simulink model "controlGPI_pos_6dof_conMI"  (R2023b)
settings: Solver=ode45  StartTime=0.0  StopTime=tsim  FixedStep=1e-4  MaxStep=tstep
undefined symbols (not defined in the file): contr_robot_params, ddq, dq, MI_Contr1, MI_Contr2, MI_Contr3, MI_Contr4, MI_Contr5, MI_Contr6, MI_motor1, MI_motor2, MI_motor3, MI_motor4, MI_motor5, MI_motor6, ndof, NN_Bspline_params, NN_RBF_params, nn_select, ns, Pc, q0, q_cero, q_eq, robot_params, sigbuilder_block, t_qeq_init, t_tr_init, t_trtr, tau_L, tau_L_mags, tr_muestra, tr_ref, Wc, Zc
libraries: mcbcontrolslib x12, spsRMSLib x12, simulink x2
(part 4 of 4)

== system controlGPI_pos_6dof_conMI/Actuadores (Motores de inducción)/MI3 + PBC Torque Controller/Controlador PBC/Ley de control ==
  i_Sref : Inport
  d_iSref : Inport  Port=2
  psi_Rref : Inport  Port=3
  w_R : Inport  Port=4
  e_iS : Inport  Port=5
  Bus Selector : BusSelector  OutputSignals=epsilon_KiS
  K_iS : MATLAB Function  TreatAsAtomicUnit=on
  Ley de control : MATLAB Function  TreatAsAtomicUnit=on
  Scope17 : Scope
  U_S : Outport
  wires:
  [K_iS] -> Ley de control/7(Ki_s)
  d_iSref/1 -> Ley de control/3(d_iSref)
  psi_Rref/1 -> Ley de control/4(psi_Rref)
  i_Sref/1 -> Ley de control/2(i_Sref)
  Ley de control/1(u_S) -> U_S/1
  w_R/1 -> [w_R], Ley de control/5(w_R)
  e_iS/1 -> Ley de control/6(e_is)
  Bus Selector/1 -> K_iS/3(epsilon)  "<epsilon_KiS>"
  K_iS/1(K_iS) -> Scope17/1, [K_iS]
  [w_R] -> K_iS/2(w_R)
  [MI_motor_params] -> Ley de control/1(MI_motor_params)
  [MI_motor_params] -> K_iS/1(MI_motor_params)
  [PBC_params] -> Bus Selector/1

== system controlGPI_pos_6dof_conMI/Actuadores (Motores de inducción)/MI3 + PBC Torque Controller/Controlador PBC/Rampa+Ret ==
  Demux : Demux  Tag=STV Demux  Outputs=1
      settings: DisplayOption=none
  FromWs : FromWorkspace  Tag=STV FromWs  VariableName=tuvar
      SigBuilderData=|
      | common.afterFinalStr = 'Extrapolate'
      | common.sampleTime = 0
      | dataSet.timeRange = [0 20]
      | dataSet.name = 'Group 1'
      | sbobj.Groups.Name = 'Group 1'
      | sbobj.Groups.Signals.Name = 'Signal 1'
      | sbobj.Groups.Signals.XData = [0 0.5 1 20]
      | sbobj.Groups.Signals.YData = [0 0 0.64 0.64]
      | sbobj.Groups.TimeRange = [0 20]
  Signal 1 : Outport  Tag=STV Outport
  wires:
  Demux/1 -> Signal 1/1
  FromWs/1 -> Demux/1

== system controlGPI_pos_6dof_conMI/Actuadores (Motores de inducción)/MI3 + PBC Torque Controller/Controlador PBC/derivada Corrientes deseadas ==
  psi_Rref : Inport
  dpsi_Rref : Inport  Port=2
  psi_Rmagref : Inport  Port=3
  dpsi_Rmagref : Inport  Port=4
  ddpsi_Rmagref : Inport  Port=5
  tau_Rref : Inport  Port=6
  dtau_Rref : Inport  Port=7
  Scope10 : Scope
  derivada Corrientes deseadas : MATLAB Function  TreatAsAtomicUnit=on
  d_iSref : Outport
  wires:
  dpsi_Rref/1 -> derivada Corrientes deseadas/3(dpsi_Rref)
  tau_Rref/1 -> derivada Corrientes deseadas/7(tau_Rref)
  dtau_Rref/1 -> derivada Corrientes deseadas/8(dtau_Rref)
  dpsi_Rmagref/1 -> derivada Corrientes deseadas/5(dpsi_Rmagref)
  derivada Corrientes deseadas/1(d_iSref) -> Scope10/1, d_iSref/1
  psi_Rmagref/1 -> derivada Corrientes deseadas/4(psi_Rmagref)
  psi_Rref/1 -> derivada Corrientes deseadas/2(psi_Rref)
  ddpsi_Rmagref/1 -> derivada Corrientes deseadas/6(ddpsi_Rmagref)
  [MI_motor_params] -> derivada Corrientes deseadas/1(MI_motor_params)

== system controlGPI_pos_6dof_conMI/Actuadores (Motores de inducción)/MI4 + PBC Torque Controller/Controlador PBC/2 a 2(1) ==
  In1 : Inport
  In2 : Inport  Port=2
  Demux1 : Demux  Outputs=2
  Demux2 : Demux  Outputs=2
  Mux : Mux  Inputs=2
  Mux1 : Mux  Inputs=2
  Out1 : Outport
  Out2 : Outport  Port=2
  wires:
  Demux2/1 -> Mux/2
  Mux/1 -> Out1/1
  In2/1 -> Demux2/1
  In1/1 -> Demux1/1
  Demux1/1 -> Mux/1
  Demux1/2 -> Mux1/1
  Mux1/1 -> Out2/1
  Demux2/2 -> Mux1/2

== system controlGPI_pos_6dof_conMI/Actuadores (Motores de inducción)/MI4 + PBC Torque Controller/Controlador PBC/Corrientes y Flujos deseados ==
  w_R : Inport
  psi_Rref : Inport  Port=2
  tau_Rref : Inport  Port=3
  psi_Rmagref : Inport  Port=4
  dpsi_Rmagref1 : Inport  Port=5
  Corrientes/Flujos deseados : MATLAB Function  TreatAsAtomicUnit=on
  i_Sref : Outport
  dpsi_Rref : Outport  Port=2
  wires:
  tau_Rref/1 -> Corrientes/Flujos deseados/4(tau_Rref)
  Corrientes/Flujos deseados/1(i_Sref) -> i_Sref/1
  psi_Rref/1 -> Corrientes/Flujos deseados/3(psi_Rref)
  w_R/1 -> Corrientes/Flujos deseados/2(w_R)
  Corrientes/Flujos deseados/2(dpsi_Rref) -> dpsi_Rref/1
  psi_Rmagref/1 -> Corrientes/Flujos deseados/5(psi_Rmagref)
  dpsi_Rmagref1/1 -> Corrientes/Flujos deseados/6(dpsi_Rmagref)
  [MI_motor_params] -> Corrientes/Flujos deseados/1(MI_motor_params)

== system controlGPI_pos_6dof_conMI/Actuadores (Motores de inducción)/MI4 + PBC Torque Controller/Controlador PBC/Ley de control ==
  i_Sref : Inport
  d_iSref : Inport  Port=2
  psi_Rref : Inport  Port=3
  w_R : Inport  Port=4
  e_iS : Inport  Port=5
  Bus Selector : BusSelector  OutputSignals=epsilon_KiS
  K_iS : MATLAB Function  TreatAsAtomicUnit=on
  Ley de control : MATLAB Function  TreatAsAtomicUnit=on
  Scope17 : Scope
  U_S : Outport
  wires:
  [K_iS] -> Ley de control/7(Ki_s)
  d_iSref/1 -> Ley de control/3(d_iSref)
  psi_Rref/1 -> Ley de control/4(psi_Rref)
  i_Sref/1 -> Ley de control/2(i_Sref)
  Ley de control/1(u_S) -> U_S/1
  w_R/1 -> [w_R], Ley de control/5(w_R)
  e_iS/1 -> Ley de control/6(e_is)
  Bus Selector/1 -> K_iS/3(epsilon)  "<epsilon_KiS>"
  K_iS/1(K_iS) -> Scope17/1, [K_iS]
  [w_R] -> K_iS/2(w_R)
  [MI_motor_params] -> Ley de control/1(MI_motor_params)
  [MI_motor_params] -> K_iS/1(MI_motor_params)
  [PBC_params] -> Bus Selector/1

== system controlGPI_pos_6dof_conMI/Actuadores (Motores de inducción)/MI4 + PBC Torque Controller/Controlador PBC/Rampa+Ret ==
  Demux : Demux  Tag=STV Demux  Outputs=1
      settings: DisplayOption=none
  FromWs : FromWorkspace  Tag=STV FromWs  VariableName=tuvar
      SigBuilderData=|
      | common.afterFinalStr = 'Extrapolate'
      | common.sampleTime = 0
      | dataSet.timeRange = [0 20]
      | dataSet.name = 'Group 1'
      | sbobj.Groups.Name = 'Group 1'
      | sbobj.Groups.Signals.Name = 'Signal 1'
      | sbobj.Groups.Signals.XData = [0 0.5 1 20]
      | sbobj.Groups.Signals.YData = [0 0 0.64 0.64]
      | sbobj.Groups.TimeRange = [0 20]
  Signal 1 : Outport  Tag=STV Outport
  wires:
  Demux/1 -> Signal 1/1
  FromWs/1 -> Demux/1

== system controlGPI_pos_6dof_conMI/Actuadores (Motores de inducción)/MI4 + PBC Torque Controller/Controlador PBC/derivada Corrientes deseadas ==
  psi_Rref : Inport
  dpsi_Rref : Inport  Port=2
  psi_Rmagref : Inport  Port=3
  dpsi_Rmagref : Inport  Port=4
  ddpsi_Rmagref : Inport  Port=5
  tau_Rref : Inport  Port=6
  dtau_Rref : Inport  Port=7
  Scope10 : Scope
  derivada Corrientes deseadas : MATLAB Function  TreatAsAtomicUnit=on
  d_iSref : Outport
  wires:
  dpsi_Rref/1 -> derivada Corrientes deseadas/3(dpsi_Rref)
  tau_Rref/1 -> derivada Corrientes deseadas/7(tau_Rref)
  dtau_Rref/1 -> derivada Corrientes deseadas/8(dtau_Rref)
  dpsi_Rmagref/1 -> derivada Corrientes deseadas/5(dpsi_Rmagref)
  derivada Corrientes deseadas/1(d_iSref) -> Scope10/1, d_iSref/1
  psi_Rmagref/1 -> derivada Corrientes deseadas/4(psi_Rmagref)
  psi_Rref/1 -> derivada Corrientes deseadas/2(psi_Rref)
  ddpsi_Rmagref/1 -> derivada Corrientes deseadas/6(ddpsi_Rmagref)
  [MI_motor_params] -> derivada Corrientes deseadas/1(MI_motor_params)

== system controlGPI_pos_6dof_conMI/Actuadores (Motores de inducción)/MI5 + PBC Torque Controller/Controlador PBC/2 a 2(1) ==
  In1 : Inport
  In2 : Inport  Port=2
  Demux1 : Demux  Outputs=2
  Demux2 : Demux  Outputs=2
  Mux : Mux  Inputs=2
  Mux1 : Mux  Inputs=2
  Out1 : Outport
  Out2 : Outport  Port=2
  wires:
  Demux2/1 -> Mux/2
  Mux/1 -> Out1/1
  In2/1 -> Demux2/1
  In1/1 -> Demux1/1
  Demux1/1 -> Mux/1
  Demux1/2 -> Mux1/1
  Mux1/1 -> Out2/1
  Demux2/2 -> Mux1/2

== system controlGPI_pos_6dof_conMI/Actuadores (Motores de inducción)/MI5 + PBC Torque Controller/Controlador PBC/Corrientes y Flujos deseados ==
  w_R : Inport
  psi_Rref : Inport  Port=2
  tau_Rref : Inport  Port=3
  psi_Rmagref : Inport  Port=4
  dpsi_Rmagref1 : Inport  Port=5
  Corrientes/Flujos deseados : MATLAB Function  TreatAsAtomicUnit=on
  i_Sref : Outport
  dpsi_Rref : Outport  Port=2
  wires:
  tau_Rref/1 -> Corrientes/Flujos deseados/4(tau_Rref)
  Corrientes/Flujos deseados/1(i_Sref) -> i_Sref/1
  psi_Rref/1 -> Corrientes/Flujos deseados/3(psi_Rref)
  w_R/1 -> Corrientes/Flujos deseados/2(w_R)
  Corrientes/Flujos deseados/2(dpsi_Rref) -> dpsi_Rref/1
  psi_Rmagref/1 -> Corrientes/Flujos deseados/5(psi_Rmagref)
  dpsi_Rmagref1/1 -> Corrientes/Flujos deseados/6(dpsi_Rmagref)
  [MI_motor_params] -> Corrientes/Flujos deseados/1(MI_motor_params)

== system controlGPI_pos_6dof_conMI/Actuadores (Motores de inducción)/MI5 + PBC Torque Controller/Controlador PBC/Ley de control ==
  i_Sref : Inport
  d_iSref : Inport  Port=2
  psi_Rref : Inport  Port=3
  w_R : Inport  Port=4
  e_iS : Inport  Port=5
  Bus Selector : BusSelector  OutputSignals=epsilon_KiS
  K_iS : MATLAB Function  TreatAsAtomicUnit=on
  Ley de control : MATLAB Function  TreatAsAtomicUnit=on
  Scope17 : Scope
  U_S : Outport
  wires:
  [K_iS] -> Ley de control/7(Ki_s)
  d_iSref/1 -> Ley de control/3(d_iSref)
  psi_Rref/1 -> Ley de control/4(psi_Rref)
  i_Sref/1 -> Ley de control/2(i_Sref)
  Ley de control/1(u_S) -> U_S/1
  w_R/1 -> [w_R], Ley de control/5(w_R)
  e_iS/1 -> Ley de control/6(e_is)
  Bus Selector/1 -> K_iS/3(epsilon)  "<epsilon_KiS>"
  K_iS/1(K_iS) -> Scope17/1, [K_iS]
  [w_R] -> K_iS/2(w_R)
  [MI_motor_params] -> Ley de control/1(MI_motor_params)
  [MI_motor_params] -> K_iS/1(MI_motor_params)
  [PBC_params] -> Bus Selector/1

== system controlGPI_pos_6dof_conMI/Actuadores (Motores de inducción)/MI5 + PBC Torque Controller/Controlador PBC/Rampa+Ret ==
  Demux : Demux  Tag=STV Demux  Outputs=1
      settings: DisplayOption=none
  FromWs : FromWorkspace  Tag=STV FromWs  VariableName=tuvar
      SigBuilderData=|
      | common.afterFinalStr = 'Extrapolate'
      | common.sampleTime = 0
      | dataSet.timeRange = [0 20]
      | dataSet.name = 'Group 1'
      | sbobj.Groups.Name = 'Group 1'
      | sbobj.Groups.Signals.Name = 'Signal 1'
      | sbobj.Groups.Signals.XData = [0 0.5 1 20]
      | sbobj.Groups.Signals.YData = [0 0 0.64 0.64]
      | sbobj.Groups.TimeRange = [0 20]
  Signal 1 : Outport  Tag=STV Outport
  wires:
  Demux/1 -> Signal 1/1
  FromWs/1 -> Demux/1

== system controlGPI_pos_6dof_conMI/Actuadores (Motores de inducción)/MI5 + PBC Torque Controller/Controlador PBC/derivada Corrientes deseadas ==
  psi_Rref : Inport
  dpsi_Rref : Inport  Port=2
  psi_Rmagref : Inport  Port=3
  dpsi_Rmagref : Inport  Port=4
  ddpsi_Rmagref : Inport  Port=5
  tau_Rref : Inport  Port=6
  dtau_Rref : Inport  Port=7
  Scope10 : Scope
  derivada Corrientes deseadas : MATLAB Function  TreatAsAtomicUnit=on
  d_iSref : Outport
  wires:
  dpsi_Rref/1 -> derivada Corrientes deseadas/3(dpsi_Rref)
  tau_Rref/1 -> derivada Corrientes deseadas/7(tau_Rref)
  dtau_Rref/1 -> derivada Corrientes deseadas/8(dtau_Rref)
  dpsi_Rmagref/1 -> derivada Corrientes deseadas/5(dpsi_Rmagref)
  derivada Corrientes deseadas/1(d_iSref) -> Scope10/1, d_iSref/1
  psi_Rmagref/1 -> derivada Corrientes deseadas/4(psi_Rmagref)
  psi_Rref/1 -> derivada Corrientes deseadas/2(psi_Rref)
  ddpsi_Rmagref/1 -> derivada Corrientes deseadas/6(ddpsi_Rmagref)
  [MI_motor_params] -> derivada Corrientes deseadas/1(MI_motor_params)

== system controlGPI_pos_6dof_conMI/Actuadores (Motores de inducción)/MI6 + PBC Torque Controller/Controlador PBC/2 a 2(1) ==
  In1 : Inport
  In2 : Inport  Port=2
  Demux1 : Demux  Outputs=2
  Demux2 : Demux  Outputs=2
  Mux : Mux  Inputs=2
  Mux1 : Mux  Inputs=2
  Out1 : Outport
  Out2 : Outport  Port=2
  wires:
  Demux2/1 -> Mux/2
  Mux/1 -> Out1/1
  In2/1 -> Demux2/1
  In1/1 -> Demux1/1
  Demux1/1 -> Mux/1
  Demux1/2 -> Mux1/1
  Mux1/1 -> Out2/1
  Demux2/2 -> Mux1/2

== system controlGPI_pos_6dof_conMI/Actuadores (Motores de inducción)/MI6 + PBC Torque Controller/Controlador PBC/Corrientes y Flujos deseados ==
  w_R : Inport
  psi_Rref : Inport  Port=2
  tau_Rref : Inport  Port=3
  psi_Rmagref : Inport  Port=4
  dpsi_Rmagref1 : Inport  Port=5
  Corrientes/Flujos deseados : MATLAB Function  TreatAsAtomicUnit=on
  i_Sref : Outport
  dpsi_Rref : Outport  Port=2
  wires:
  tau_Rref/1 -> Corrientes/Flujos deseados/4(tau_Rref)
  Corrientes/Flujos deseados/1(i_Sref) -> i_Sref/1
  psi_Rref/1 -> Corrientes/Flujos deseados/3(psi_Rref)
  w_R/1 -> Corrientes/Flujos deseados/2(w_R)
  Corrientes/Flujos deseados/2(dpsi_Rref) -> dpsi_Rref/1
  psi_Rmagref/1 -> Corrientes/Flujos deseados/5(psi_Rmagref)
  dpsi_Rmagref1/1 -> Corrientes/Flujos deseados/6(dpsi_Rmagref)
  [MI_motor_params] -> Corrientes/Flujos deseados/1(MI_motor_params)

== system controlGPI_pos_6dof_conMI/Actuadores (Motores de inducción)/MI6 + PBC Torque Controller/Controlador PBC/Ley de control ==
  i_Sref : Inport
  d_iSref : Inport  Port=2
  psi_Rref : Inport  Port=3
  w_R : Inport  Port=4
  e_iS : Inport  Port=5
  Bus Selector : BusSelector  OutputSignals=epsilon_KiS
  K_iS : MATLAB Function  TreatAsAtomicUnit=on
  Ley de control : MATLAB Function  TreatAsAtomicUnit=on
  Scope17 : Scope
  U_S : Outport
  wires:
  [K_iS] -> Ley de control/7(Ki_s)
  d_iSref/1 -> Ley de control/3(d_iSref)
  psi_Rref/1 -> Ley de control/4(psi_Rref)
  i_Sref/1 -> Ley de control/2(i_Sref)
  Ley de control/1(u_S) -> U_S/1
  w_R/1 -> [w_R], Ley de control/5(w_R)
  e_iS/1 -> Ley de control/6(e_is)
  Bus Selector/1 -> K_iS/3(epsilon)  "<epsilon_KiS>"
  K_iS/1(K_iS) -> Scope17/1, [K_iS]
  [w_R] -> K_iS/2(w_R)
  [MI_motor_params] -> Ley de control/1(MI_motor_params)
  [MI_motor_params] -> K_iS/1(MI_motor_params)
  [PBC_params] -> Bus Selector/1

== system controlGPI_pos_6dof_conMI/Actuadores (Motores de inducción)/MI6 + PBC Torque Controller/Controlador PBC/Rampa+Ret ==
  Demux : Demux  Tag=STV Demux  Outputs=1
      settings: DisplayOption=none
  FromWs : FromWorkspace  Tag=STV FromWs  VariableName=tuvar
      SigBuilderData=|
      | common.afterFinalStr = 'Extrapolate'
      | common.sampleTime = 0
      | dataSet.timeRange = [0 20]
      | dataSet.name = 'Group 1'
      | sbobj.Groups.Name = 'Group 1'
      | sbobj.Groups.Signals.Name = 'Signal 1'
      | sbobj.Groups.Signals.XData = [0 0.5 1 20]
      | sbobj.Groups.Signals.YData = [0 0 0.64 0.64]
      | sbobj.Groups.TimeRange = [0 20]
  Signal 1 : Outport  Tag=STV Outport
  wires:
  Demux/1 -> Signal 1/1
  FromWs/1 -> Demux/1

== system controlGPI_pos_6dof_conMI/Actuadores (Motores de inducción)/MI6 + PBC Torque Controller/Controlador PBC/derivada Corrientes deseadas ==
  psi_Rref : Inport
  dpsi_Rref : Inport  Port=2
  psi_Rmagref : Inport  Port=3
  dpsi_Rmagref : Inport  Port=4
  ddpsi_Rmagref : Inport  Port=5
  tau_Rref : Inport  Port=6
  dtau_Rref : Inport  Port=7
  Scope10 : Scope
  derivada Corrientes deseadas : MATLAB Function  TreatAsAtomicUnit=on
  d_iSref : Outport
  wires:
  dpsi_Rref/1 -> derivada Corrientes deseadas/3(dpsi_Rref)
  tau_Rref/1 -> derivada Corrientes deseadas/7(tau_Rref)
  dtau_Rref/1 -> derivada Corrientes deseadas/8(dtau_Rref)
  dpsi_Rmagref/1 -> derivada Corrientes deseadas/5(dpsi_Rmagref)
  derivada Corrientes deseadas/1(d_iSref) -> Scope10/1, d_iSref/1
  psi_Rmagref/1 -> derivada Corrientes deseadas/4(psi_Rmagref)
  psi_Rref/1 -> derivada Corrientes deseadas/2(psi_Rref)
  ddpsi_Rmagref/1 -> derivada Corrientes deseadas/6(ddpsi_Rmagref)
  [MI_motor_params] -> derivada Corrientes deseadas/1(MI_motor_params)

== matlab function controlGPI_pos_6dof_conMI/ControladorGPI + NN/Ley de control ==
  data: robot_din input; v output size=[6,1]; eqB5 input size=[6,1]; eqB4 input size=[6,1]; eqB3 input size=[6,1]; eqB2 input size=[6,1]; eqB1 input size=[6,1]; tau_R output size=[6,1]
function [v,tau_R] = fcn(robot_din,eqB5,eqB4,eqB3,eqB2,eqB1)

D = robot_din.D;

v = - eqB5 - eqB4 - eqB3 - eqB2 - eqB1;

tau_R = D*v;

== matlab function controlGPI_pos_6dof_conMI/ControladorGPI + NN/Matriz de parámetros B ==
  data: B5 output size=[6,1]; B4 output size=[6,1]; B3 output size=[6,1]; B2 output size=[6,1]; Zc input size=[6,1]; B1 output size=[6,1]; Wc input size=[6,1]; Pc input size=[6,1]
function [B5,B4,B3,B2,B1] = fcn(Zc,Wc,Pc)

B = zeros(6,6);

B(:,1) = Wc.^4.*Pc;
B(:,2) = 4*Wc.^3.*Zc.*Pc + Wc.^4;
B(:,3) = 4*Wc.^3.*Zc + 4*Wc.^2.*Zc.^2.*Pc + 2.*Wc.^2.*Pc;
B(:,4) = 2*Wc.^2 + 4*Wc.^2.*Zc.^2 + 4*Wc.*Zc.*Pc;
B(:,5) = 4*Wc.*Zc + Pc;
% B(:,6) = ones(3,6);

B1 = B(:,1);
B2 = B(:,2);
B3 = B(:,3);
B4 = B(:,4);
B5 = B(:,5);
% B6 = B(:,6);

== matlab function controlGPI_pos_6dof_conMI/ControladorGPI + NN/Red neuronal/B-Spline NNs/Red Neuronal B-spline ==
  data: NN_Bspline_params input; e_q input size=[6,1]; Wc output size=[6,1]; Zc output size=[6,1]; Pc output size=[6,1]; e_px input size=[6,1]; e_py input size=[6,1]; e_pz input size=[6,1]; newweightsWc output; newweightsZc output; newweightsPc output; weightsWc input; weightsZc input; weightsPc input
function [Wc, Zc, Pc, newweightsWc, newweightsZc, newweightsPc]   = BSpline_NN(NN_Bspline_params,e_q,e_px,e_py,e_pz,weightsWc,weightsZc,weightsPc)

deltaWc = NN_Bspline_params.delta.deltaWc;
deltaZc = NN_Bspline_params.delta.deltaZc;
deltaPc = NN_Bspline_params.delta.deltaPc;

lambdaWc = NN_Bspline_params.lambda.lambdaWc;
lambdaZc = NN_Bspline_params.lambda.lambdaZc;
lambdaPc = NN_Bspline_params.lambda.lambdaPc;

if NN_Bspline_params.num_inputs == 1
    nn_inputs = e_q;
elseif NN_Bspline_params.num_inputs == 4
    nn_inputs = [e_q,e_px,e_py,e_pz];
else
    nn_inputs = e_q;
end

delta = [deltaWc;
         deltaZc;
         deltaPc];

lambda = cat(1,lambdaWc,lambdaZc,lambdaPc);
weights = cat(1,weightsWc,weightsZc,weightsPc);

[newparams,newweights] = NN_Bspline.Gradient_Descent(delta,weights,lambda,nn_inputs);

Wc = newparams(1,:)';
Zc = newparams(2,:)';
Pc = newparams(3,:)';

newweightsWc = newweights(1,:,:);
newweightsZc = newweights(2,:,:);
newweightsPc = newweights(3,:,:);

end

== matlab function controlGPI_pos_6dof_conMI/ControladorGPI + NN/Red neuronal/RBF NNs/Red Neuronal RBF ==
  data: NN_RBF_params input; e_q input size=[6,1]; Wc output size=[6,1]; Zc output size=[6,1]; Pc output size=[6,1]; e_px input size=[6,1]; e_py input size=[6,1]; e_pz input size=[6,1]; weightsWc output; weightsZc output; weightsPc output; weightsWc input; weightsZc input; weightsPc input
function [Wc, Zc, Pc, weightsWc, weightsZc, weightsPc] = RBF_NN(NN_RBF_params,e_q,e_px,e_py,e_pz, weightsWc, weightsZc, weightsPc)

%k = NN_RBF_params.rbf_params.k;
centers = NN_RBF_params.rbf_params.C';
radius = NN_RBF_params.rbf_params.sigma;

deltaWc = NN_RBF_params.delta.deltaWc;
deltaZc = NN_RBF_params.delta.deltaZc;
deltaPc = NN_RBF_params.delta.deltaPc;

if NN_RBF_params.num_inputs == 1
    NNRBF_inputs = e_q;
elseif NN_RBF_params.num_inputs == 4
    NNRBF_inputs = [e_q,e_px,e_py,e_pz];
else
    NNRBF_inputs = e_q;
end

delta = [deltaWc;
         deltaZc;
         deltaPc];

weights = cat(1,weightsWc,weightsZc,weightsPc);

[newparams,newweights] = NN_RBF.Gradient_Descent(delta,weights,centers,radius,NNRBF_inputs);

Wc = newparams(1,:)';
Zc = newparams(2,:)';
Pc = newparams(3,:)';

weightsWc = newweights(1,:,:);
weightsZc = newweights(2,:,:);
weightsPc = newweights(3,:,:);

end

== matlab function controlGPI_pos_6dof_conMI/Perfil torque de carga tau_L/If Action Subsystem/Polinomio 7mo orden sen ==
  data: t input; perfil_params input; qpol output; vpol output; apol output; jpol output
function [qpol,vpol,apol,jpol] = fcn(t,perfil_params)

%Trayectoria de referencia

q0 = 0;
q1 = perfil_params.senoidal.amplitud;

% v0 = perfil_params.polinomio7.vel.inicial;
% v1 = perfil_params.polinomio7.vel.final;
% 
% ac0 = perfil_params.polinomio7.acel.inicial;
% ac1 = perfil_params.polinomio7.acel.final;
% 
% j0 = perfil_params.polinomio7.jerk.inicial;
% j1 = perfil_params.polinomio7.jerk.inicial;

if perfil_params.senoidal.tiempo_inicio-1>0
    t0 = perfil_params.senoidal.tiempo_inicio-1;
else
    t0 = 0;
end
t1 = perfil_params.senoidal.tiempo_inicio;

% Coeficientes de un polinomio de 7mo grado
[qpol,vpol,apol,jpol] = pol7(t,q1,q0,t0,t1);

== matlab function controlGPI_pos_6dof_conMI/Perfil torque de carga tau_L/If Action Subsystem4/Polinomio 7mo orden tau_L ==
  data: t input; perfil_params input; qpol output; vpol output; apol output; jpol output
function [qpol,vpol,apol,jpol] = fcn(t,perfil_params)

%Trayectoria de referencia

q0 = perfil_params.polinomio7.pos.inicial;
q1 = perfil_params.polinomio7.pos.final;

% v0 = perfil_params.polinomio7.vel.inicial;
% v1 = perfil_params.polinomio7.vel.final;
% 
% ac0 = perfil_params.polinomio7.acel.inicial;
% ac1 = perfil_params.polinomio7.acel.final;
% 
% j0 = perfil_params.polinomio7.jerk.inicial;
% j1 = perfil_params.polinomio7.jerk.inicial;

t0 = perfil_params.polinomio7.tiempo.inicial;
t1 = perfil_params.polinomio7.tiempo.final;

% Coeficientes de un polinomio de 7mo grado
[qpol,vpol,apol,jpol] = pol7(t,q0,q1,t0,t1);

== matlab function controlGPI_pos_6dof_conMI/Perfil torque de carga tau_L/If Action Subsystem7/Trayectoria 15 segmentos ==
  data: t input size=1; q output size=1; perfil_params input
function q = fcn(t,perfil_params)

q0 = perfil_params.tr15segs.pos.inicial;
q1 = perfil_params.tr15segs.pos.final;

t0 = perfil_params.tr15segs.tiempo.inicial;

vel_path = perfil_params.tr15segs.vel_path;
acel_path = perfil_params.tr15segs.acel_path;
snap_path = perfil_params.tr15segs.snap_path;

dist = norm(q1-q0);
num_steps = 1000;




[interq,T] = pol15segs.bounded_tr(dist,num_steps,vel_path,acel_path,snap_path,0);

tstep = T/num_steps;
t1 = t0 + T;
t_tr = (t0:tstep:t1)';


[~,idt] = min(t_tr-t);
dire = (q1 - q0)/dist;
q = q0 + dire*interq(idt);

== matlab function controlGPI_pos_6dof_conMI/ISCI ==
  data: tau input; ISCI output
function ISCI = fcn(tau)

ISCI = tau.^2;

== matlab function controlGPI_pos_6dof_conMI/Perfil torque de carga tau_L/If Action Subsystem6/Polinomio 7mo orden timeseries ==
  data: t input; qpol output; vpol output; apol output; jpol output
function [qpol,vpol,apol,jpol] = fcn(t)

q0 = 0;
q1 = 1;

t0 = 0.5;
t1 = 1;

%Trayectoria de referencia

% Coeficientes de un polinomio de 7mo grado
[qpol,vpol,apol,jpol] = pol7(t,q0,q1,t0,t1);

== matlab function controlGPI_pos_6dof_conMI/Actuadores (Motores de inducción)/MI3 + PBC Torque Controller/Calculo de Potencia eléctrica/ab0 - ABC1 ==
  data: BPu input size=[2,1]; u output size=[3,1]
function u = fcn(BPu)

BPu = vertcat(BPu,0);

% Power invariant
BP = transforms.Clarke_transform(1);

u = BP^-1*BPu;

== matlab function controlGPI_pos_6dof_conMI/Perfil torque de carga tau_L/If Action Subsystem5/Tren de esca ==
  data: t input; q output; perfil_params input
function q = fcn(t,perfil_params)

q = Perfil_trayectoria.trEsca(t,perfil_params);

== matlab function controlGPI_pos_6dof_conMI/ITAE ==
  data: t input; ITAE output; eq input
function ITAE = fcn(t,eq)

ITAE = t.*abs(eq);

== matlab function controlGPI_pos_6dof_conMI/Actuadores (Motores de inducción)/MI2 + PBC Torque Controller/Calculo de Potencia eléctrica/ab0 - ABC ==
  data: BPu input size=[2,1]; u output size=[3,1]
function u = fcn(BPu)

BPu = vertcat(BPu,0);

% Power invariant
BP = transforms.Clarke_transform(1);

u = BP^-1*BPu;

== matlab function controlGPI_pos_6dof_conMI/Actuadores (Motores de inducción)/MI2 + PBC Torque Controller/Calculo de Potencia eléctrica/ab0 - ABC1 ==
  data: BPu input size=[2,1]; u output size=[3,1]
function u = fcn(BPu)

BPu = vertcat(BPu,0);

% Power invariant
BP = transforms.Clarke_transform(1);

u = BP^-1*BPu;

== matlab function controlGPI_pos_6dof_conMI/Actuadores (Motores de inducción)/MI2 + PBC Torque Controller/Controlador PBC/Corrientes y Flujos deseados/Corrientes//Flujos deseados ==
  data: MI_motor_params input; w_R input; i_Sref output size=[2 1]; psi_Rref input size=[2,1]; tau_Rref input; psi_Rmagref input; dpsi_Rmagref input; dpsi_Rref output size=[2,1]
function [i_Sref,dpsi_Rref] = fcn(MI_motor_params,w_R,psi_Rref,tau_Rref,psi_Rmagref,dpsi_Rmagref)

i_Sref = PBC_Torque_Controller.i_Sref(MI_motor_params,psi_Rref,tau_Rref,psi_Rmagref,dpsi_Rmagref);
dpsi_Rref = PBC_Torque_Controller.dpsi_Ref(MI_motor_params,w_R,psi_Rref,tau_Rref,psi_Rmagref,dpsi_Rmagref);

== matlab function controlGPI_pos_6dof_conMI/Actuadores (Motores de inducción)/MI2 + PBC Torque Controller/Controlador PBC/Ley de control/K_iS ==
  data: MI_motor_params input; w_R input; epsilon input; K_iS output
function K_iS = fcn(MI_motor_params,w_R,epsilon)

K_iS = PBC_Torque_Controller.K_iS(MI_motor_params,w_R,epsilon);

== matlab function controlGPI_pos_6dof_conMI/Modelo robot manipulador (Dinámica directa)/Dinámica directa ==
  data: robot_params input; q input; ddq output size=[6,1]; dq input size=[6,1]; tau_R input size=[6,1]; tau_L input size=[6,1]
function ddq = fcn(robot_params,q,dq,tau_R,tau_L)

robot_din = robot_dinm.din_6dof(robot_params,q,dq);

D = robot_din.D;
C = robot_din.C;
G = robot_din.G;
g = robot_din.g;

ddq = D^-1*(-C*dq-G*g+(tau_R-tau_L));

== matlab function controlGPI_pos_6dof_conMI/Actuadores (Motores de inducción)/MI3 + PBC Torque Controller/Controlador PBC/Corrientes y Flujos deseados/Corrientes//Flujos deseados ==
  data: MI_motor_params input; w_R input; i_Sref output size=[2 1]; psi_Rref input size=[2,1]; tau_Rref input; psi_Rmagref input; dpsi_Rmagref input; dpsi_Rref output size=[2,1]
function [i_Sref,dpsi_Rref] = fcn(MI_motor_params,w_R,psi_Rref,tau_Rref,psi_Rmagref,dpsi_Rmagref)

i_Sref = PBC_Torque_Controller.i_Sref(MI_motor_params,psi_Rref,tau_Rref,psi_Rmagref,dpsi_Rmagref);
dpsi_Rref = PBC_Torque_Controller.dpsi_Ref(MI_motor_params,w_R,psi_Rref,tau_Rref,psi_Rmagref,dpsi_Rmagref);

== matlab function controlGPI_pos_6dof_conMI/Actuadores (Motores de inducción)/MI3 + PBC Torque Controller/Controlador PBC/Ley de control/K_iS ==
  data: MI_motor_params input; w_R input; epsilon input; K_iS output
function K_iS = fcn(MI_motor_params,w_R,epsilon)

K_iS = PBC_Torque_Controller.K_iS(MI_motor_params,w_R,epsilon);

== matlab function controlGPI_pos_6dof_conMI/Actuadores (Motores de inducción)/MI2 + PBC Torque Controller/Controlador PBC/Ley de control/Ley de control ==
  data: MI_motor_params input; i_Sref input size=[2,1]; d_iSref input size=[2,1]; u_S output size=[2 1]; psi_Rref input size=[2,1]; w_R input; e_is input; Ki_s input
function u_S = fcn(MI_motor_params,i_Sref,d_iSref,psi_Rref,w_R,e_is,Ki_s)

u_S = PBC_Torque_Controller.ley_control_uS(MI_motor_params,i_Sref,d_iSref,psi_Rref,w_R,e_is,Ki_s);

== matlab function controlGPI_pos_6dof_conMI/Actuadores (Motores de inducción)/MI1 + PBC Torque Controller/Controlador PBC/Corrientes y Flujos deseados/Corrientes//Flujos deseados ==
  data: MI_motor_params input; w_R input; i_Sref output size=[2 1]; psi_Rref input size=[2,1]; tau_Rref input; psi_Rmagref input; dpsi_Rmagref input; dpsi_Rref output size=[2,1]
function [i_Sref,dpsi_Rref] = fcn(MI_motor_params,w_R,psi_Rref,tau_Rref,psi_Rmagref,dpsi_Rmagref)

i_Sref = PBC_Torque_Controller.i_Sref(MI_motor_params,psi_Rref,tau_Rref,psi_Rmagref,dpsi_Rmagref);
dpsi_Rref = PBC_Torque_Controller.dpsi_Ref(MI_motor_params,w_R,psi_Rref,tau_Rref,psi_Rmagref,dpsi_Rmagref);

== matlab function controlGPI_pos_6dof_conMI/Actuadores (Motores de inducción)/MI1 + PBC Torque Controller/Controlador PBC/Ley de control/K_iS ==
  data: MI_motor_params input; w_R input; epsilon input; K_iS output
function K_iS = fcn(MI_motor_params,w_R,epsilon)

K_iS = PBC_Torque_Controller.K_iS(MI_motor_params,w_R,epsilon);

== matlab function controlGPI_pos_6dof_conMI/Trayectoria de referencia/Dinamica inversa (referencia) ==
  data: robot_params input; tau_s output size=[6,1]; q input size=[6,1]; dq input size=[6,1]; ddq input size=[6,1]
function tau_s = fcn(robot_params,q,dq,ddq)

robot_din = robot_dinm.din_6dof(robot_params,q,dq);

D = robot_din.D;
C = robot_din.C;
G = robot_din.G;
g = robot_din.g;

tau_s = D*ddq + C*dq + G*g;

== matlab function controlGPI_pos_6dof_conMI/Actuadores (Motores de inducción)/MI1 + PBC Torque Controller/Calculo de Potencia eléctrica/ab0 - ABC ==
  data: BPu input size=[2,1]; u output size=[3,1]
function u = fcn(BPu)

BPu = vertcat(BPu,0);

% Power invariant
BP = transforms.Clarke_transform(1);

u = BP^-1*BPu;

== matlab function controlGPI_pos_6dof_conMI/Actuadores (Motores de inducción)/MI1 + PBC Torque Controller/Controlador PBC/Ley de control/Ley de control ==
  data: MI_motor_params input; i_Sref input size=[2,1]; d_iSref input size=[2,1]; u_S output size=[2 1]; psi_Rref input size=[2,1]; w_R input; e_is input; Ki_s input
function u_S = fcn(MI_motor_params,i_Sref,d_iSref,psi_Rref,w_R,e_is,Ki_s)

u_S = PBC_Torque_Controller.ley_control_uS(MI_motor_params,i_Sref,d_iSref,psi_Rref,w_R,e_is,Ki_s);

== matlab function controlGPI_pos_6dof_conMI/Actuadores (Motores de inducción)/MI1 + PBC Torque Controller/Calculo de Potencia eléctrica/ab0 - ABC1 ==
  data: BPu input size=[2,1]; u output size=[3,1]
function u = fcn(BPu)

BPu = vertcat(BPu,0);

% Power invariant
BP = transforms.Clarke_transform(1);

u = BP^-1*BPu;

== matlab function controlGPI_pos_6dof_conMI/Actuadores (Motores de inducción)/MI3 + PBC Torque Controller/Controlador PBC/Ley de control/Ley de control ==
  data: MI_motor_params input; i_Sref input size=[2,1]; d_iSref input size=[2,1]; u_S output size=[2 1]; psi_Rref input size=[2,1]; w_R input; e_is input; Ki_s input
function u_S = fcn(MI_motor_params,i_Sref,d_iSref,psi_Rref,w_R,e_is,Ki_s)

u_S = PBC_Torque_Controller.ley_control_uS(MI_motor_params,i_Sref,d_iSref,psi_Rref,w_R,e_is,Ki_s);

== matlab function controlGPI_pos_6dof_conMI/Actuadores (Motores de inducción)/MI3 + PBC Torque Controller/Controlador PBC/derivada Corrientes deseadas/derivada Corrientes deseadas ==
  data: MI_motor_params input; d_iSref output size=[2 1]; psi_Rref input size=[2,1]; dpsi_Rref input size=[2,1]; psi_Rmagref input; dpsi_Rmagref input; ddpsi_Rmagref input; tau_Rref input; dtau_Rref input
function d_iSref = fcn(MI_motor_params,psi_Rref,dpsi_Rref,psi_Rmagref,dpsi_Rmagref,ddpsi_Rmagref,tau_Rref,dtau_Rref)

d_iSref = PBC_Torque_Controller.d_iSref(MI_motor_params,psi_Rref,dpsi_Rref,psi_Rmagref,dpsi_Rmagref,ddpsi_Rmagref,tau_Rref,dtau_Rref);

== matlab function controlGPI_pos_6dof_conMI/Actuadores (Motores de inducción)/MI3 + PBC Torque Controller/Modelo MI (Subsistema eléctrico)/Modelo Motor de inducción (Subsistema eléctrico) ==
  data: MI_motor_params input; di_Sab output double size=[2 1]; dpsi_Rab output double size=[2 1]; u_Sab input double size=[2 1]; i_Sab input double size=[2 1]; psi_Rab input double size=[2 1]; w_R input double size=1; tau_R output size=1; tau_L input
function [di_Sab,dpsi_Rab,tau_R] = fcn(MI_motor_params,u_Sab,i_Sab,psi_Rab,w_R,tau_L)

[di_Sab,dpsi_Rab,dw_R,tau_R] = MI_model.MI_space_state(MI_motor_params,u_Sab,i_Sab,psi_Rab,w_R,tau_L);

== matlab function controlGPI_pos_6dof_conMI/Actuadores (Motores de inducción)/MI1 + PBC Torque Controller/Controlador PBC/derivada Corrientes deseadas/derivada Corrientes deseadas ==
  data: MI_motor_params input; d_iSref output size=[2 1]; psi_Rref input size=[2,1]; dpsi_Rref input size=[2,1]; psi_Rmagref input; dpsi_Rmagref input; ddpsi_Rmagref input; tau_Rref input; dtau_Rref input
function d_iSref = fcn(MI_motor_params,psi_Rref,dpsi_Rref,psi_Rmagref,dpsi_Rmagref,ddpsi_Rmagref,tau_Rref,dtau_Rref)

d_iSref = PBC_Torque_Controller.d_iSref(MI_motor_params,psi_Rref,dpsi_Rref,psi_Rmagref,dpsi_Rmagref,ddpsi_Rmagref,tau_Rref,dtau_Rref);

== matlab function controlGPI_pos_6dof_conMI/Actuadores (Motores de inducción)/MI1 + PBC Torque Controller/Modelo MI (Subsistema eléctrico)/Modelo Motor de inducción (Subsistema eléctrico) ==
  data: MI_motor_params input; di_Sab output double size=[2 1]; dpsi_Rab output double size=[2 1]; u_Sab input double size=[2 1]; i_Sab input double size=[2 1]; psi_Rab input double size=[2 1]; w_R input double size=1; tau_R output size=1; tau_L input
function [di_Sab,dpsi_Rab,tau_R] = fcn(MI_motor_params,u_Sab,i_Sab,psi_Rab,w_R,tau_L)

[di_Sab,dpsi_Rab,dw_R,tau_R] = MI_model.MI_space_state(MI_motor_params,u_Sab,i_Sab,psi_Rab,w_R,tau_L);

== matlab function controlGPI_pos_6dof_conMI/Actuadores (Motores de inducción)/MI1 + PBC Torque Controller/Modelo MI (Subsistema eléctrico)/ab//dq ==
  data: psi_ra input; psi_Rmag output; psi_rb input; rho output
function [psi_Rmag,rho] = fcn(psi_ra,psi_rb)

psi_Rmag = sqrt(psi_ra^2+psi_rb^2);
rho = atan2(psi_rb,psi_ra);

== matlab function controlGPI_pos_6dof_conMI/Actuadores (Motores de inducción)/MI3 + PBC Torque Controller/Modelo MI (Subsistema eléctrico)/ab//dq ==
  data: psi_ra input; psi_Rmag output; psi_rb input; rho output
function [psi_Rmag,rho] = fcn(psi_ra,psi_rb)

psi_Rmag = sqrt(psi_ra^2+psi_rb^2);
rho = atan2(psi_rb,psi_ra);

== matlab function controlGPI_pos_6dof_conMI/Actuadores (Motores de inducción)/MI4 + PBC Torque Controller/Calculo de Potencia eléctrica/ab0 - ABC ==
  data: BPu input size=[2,1]; u output size=[3,1]
function u = fcn(BPu)

BPu = vertcat(BPu,0);

% Power invariant
BP = transforms.Clarke_transform(1);

u = BP^-1*BPu;

== matlab function controlGPI_pos_6dof_conMI/Actuadores (Motores de inducción)/MI4 + PBC Torque Controller/Calculo de Potencia eléctrica/ab0 - ABC1 ==
  data: BPu input size=[2,1]; u output size=[3,1]
function u = fcn(BPu)

BPu = vertcat(BPu,0);

% Power invariant
BP = transforms.Clarke_transform(1);

u = BP^-1*BPu;

== matlab function controlGPI_pos_6dof_conMI/Trayectoria de referencia/q to xyz (referencia) ==
  data: p output size=[3,6]; robot_params input; q input size=[6,1]
function p = fcn(robot_params,q)

p = robot_cin.cin_dirp_6dof(robot_params,q);

== matlab function controlGPI_pos_6dof_conMI/Trayectoria de referencia/xyz to q (referencia) ==
  data: robot_params input; q output size=[6,1]; r input size=[3,1]; dr input size=[3,1]; ddr input size=[3,1]; dq output size=[6,1]; ddq output size=[6,1]; R input size=[3,3]
function [q,dq,ddq] = fcn(robot_params,r,dr,ddr,R)

[q,dq,ddq] = robot_cin.cin_inv_6dof(robot_params,r,dr,ddr,R);

== matlab function controlGPI_pos_6dof_conMI/q to xyz (robot)/q to xyz (robot) ==
  data: p output size=[3,6]; robot_params input; q input size=[6,1]; dq input size=[6,1]; ddq input size=[6,1]; dp output size=[3,1]; ddp output size=[3,1]
function [p,dp,ddp] = fcn(robot_params,q,dq,ddq)

p = robot_cin.cin_dirp_6dof(robot_params,q);

JP = robot_cin.JP_6dof(robot_params,q);
dp = JP*dq;

dJP = robot_cin.dJP_6dof(robot_params,q,dq);
ddp = dJP*ddq;

== matlab function controlGPI_pos_6dof_conMI/Actuadores (Motores de inducción)/MI4 + PBC Torque Controller/Controlador PBC/Corrientes y Flujos deseados/Corrientes//Flujos deseados ==
  data: MI_motor_params input; w_R input; i_Sref output size=[2 1]; psi_Rref input size=[2,1]; tau_Rref input; psi_Rmagref input; dpsi_Rmagref input; dpsi_Rref output size=[2,1]
function [i_Sref,dpsi_Rref] = fcn(MI_motor_params,w_R,psi_Rref,tau_Rref,psi_Rmagref,dpsi_Rmagref)

i_Sref = PBC_Torque_Controller.i_Sref(MI_motor_params,psi_Rref,tau_Rref,psi_Rmagref,dpsi_Rmagref);
dpsi_Rref = PBC_Torque_Controller.dpsi_Ref(MI_motor_params,w_R,psi_Rref,tau_Rref,psi_Rmagref,dpsi_Rmagref);

== matlab function controlGPI_pos_6dof_conMI/Actuadores (Motores de inducción)/MI4 + PBC Torque Controller/Controlador PBC/Ley de control/K_iS ==
  data: MI_motor_params input; w_R input; epsilon input; K_iS output
function K_iS = fcn(MI_motor_params,w_R,epsilon)

K_iS = PBC_Torque_Controller.K_iS(MI_motor_params,w_R,epsilon);

== matlab function controlGPI_pos_6dof_conMI/Actuadores (Motores de inducción)/MI4 + PBC Torque Controller/Controlador PBC/Ley de control/Ley de control ==
  data: MI_motor_params input; i_Sref input size=[2,1]; d_iSref input size=[2,1]; u_S output size=[2 1]; psi_Rref input size=[2,1]; w_R input; e_is input; Ki_s input
function u_S = fcn(MI_motor_params,i_Sref,d_iSref,psi_Rref,w_R,e_is,Ki_s)

u_S = PBC_Torque_Controller.ley_control_uS(MI_motor_params,i_Sref,d_iSref,psi_Rref,w_R,e_is,Ki_s);

== matlab function controlGPI_pos_6dof_conMI/Actuadores (Motores de inducción)/MI4 + PBC Torque Controller/Controlador PBC/derivada Corrientes deseadas/derivada Corrientes deseadas ==
  data: MI_motor_params input; d_iSref output size=[2 1]; psi_Rref input size=[2,1]; dpsi_Rref input size=[2,1]; psi_Rmagref input; dpsi_Rmagref input; ddpsi_Rmagref input; tau_Rref input; dtau_Rref input
function d_iSref = fcn(MI_motor_params,psi_Rref,dpsi_Rref,psi_Rmagref,dpsi_Rmagref,ddpsi_Rmagref,tau_Rref,dtau_Rref)

d_iSref = PBC_Torque_Controller.d_iSref(MI_motor_params,psi_Rref,dpsi_Rref,psi_Rmagref,dpsi_Rmagref,ddpsi_Rmagref,tau_Rref,dtau_Rref);

== matlab function controlGPI_pos_6dof_conMI/Actuadores (Motores de inducción)/MI4 + PBC Torque Controller/Modelo MI (Subsistema eléctrico)/Modelo Motor de inducción (Subsistema eléctrico) ==
  data: MI_motor_params input; di_Sab output double size=[2 1]; dpsi_Rab output double size=[2 1]; u_Sab input double size=[2 1]; i_Sab input double size=[2 1]; psi_Rab input double size=[2 1]; w_R input double size=1; tau_R output size=1; tau_L input
function [di_Sab,dpsi_Rab,tau_R] = fcn(MI_motor_params,u_Sab,i_Sab,psi_Rab,w_R,tau_L)

[di_Sab,dpsi_Rab,dw_R,tau_R] = MI_model.MI_space_state(MI_motor_params,u_Sab,i_Sab,psi_Rab,w_R,tau_L);

== matlab function controlGPI_pos_6dof_conMI/Actuadores (Motores de inducción)/MI4 + PBC Torque Controller/Modelo MI (Subsistema eléctrico)/ab//dq ==
  data: psi_ra input; psi_Rmag output; psi_rb input; rho output
function [psi_Rmag,rho] = fcn(psi_ra,psi_rb)

psi_Rmag = sqrt(psi_ra^2+psi_rb^2);
rho = atan2(psi_rb,psi_ra);

== matlab function controlGPI_pos_6dof_conMI/Actuadores (Motores de inducción)/MI5 + PBC Torque Controller/Calculo de Potencia eléctrica/ab0 - ABC ==
  data: BPu input size=[2,1]; u output size=[3,1]
function u = fcn(BPu)

BPu = vertcat(BPu,0);

% Power invariant
BP = transforms.Clarke_transform(1);

u = BP^-1*BPu;

== matlab function controlGPI_pos_6dof_conMI/Actuadores (Motores de inducción)/MI5 + PBC Torque Controller/Calculo de Potencia eléctrica/ab0 - ABC1 ==
  data: BPu input size=[2,1]; u output size=[3,1]
function u = fcn(BPu)

BPu = vertcat(BPu,0);

% Power invariant
BP = transforms.Clarke_transform(1);

u = BP^-1*BPu;

== matlab function controlGPI_pos_6dof_conMI/Actuadores (Motores de inducción)/MI5 + PBC Torque Controller/Controlador PBC/Corrientes y Flujos deseados/Corrientes//Flujos deseados ==
  data: MI_motor_params input; w_R input; i_Sref output size=[2 1]; psi_Rref input size=[2,1]; tau_Rref input; psi_Rmagref input; dpsi_Rmagref input; dpsi_Rref output size=[2,1]
function [i_Sref,dpsi_Rref] = fcn(MI_motor_params,w_R,psi_Rref,tau_Rref,psi_Rmagref,dpsi_Rmagref)

i_Sref = PBC_Torque_Controller.i_Sref(MI_motor_params,psi_Rref,tau_Rref,psi_Rmagref,dpsi_Rmagref);
dpsi_Rref = PBC_Torque_Controller.dpsi_Ref(MI_motor_params,w_R,psi_Rref,tau_Rref,psi_Rmagref,dpsi_Rmagref);

== matlab function controlGPI_pos_6dof_conMI/Actuadores (Motores de inducción)/MI5 + PBC Torque Controller/Controlador PBC/Ley de control/K_iS ==
  data: MI_motor_params input; w_R input; epsilon input; K_iS output
function K_iS = fcn(MI_motor_params,w_R,epsilon)

K_iS = PBC_Torque_Controller.K_iS(MI_motor_params,w_R,epsilon);

== matlab function controlGPI_pos_6dof_conMI/Actuadores (Motores de inducción)/MI5 + PBC Torque Controller/Controlador PBC/Ley de control/Ley de control ==
  data: MI_motor_params input; i_Sref input size=[2,1]; d_iSref input size=[2,1]; u_S output size=[2 1]; psi_Rref input size=[2,1]; w_R input; e_is input; Ki_s input
function u_S = fcn(MI_motor_params,i_Sref,d_iSref,psi_Rref,w_R,e_is,Ki_s)

u_S = PBC_Torque_Controller.ley_control_uS(MI_motor_params,i_Sref,d_iSref,psi_Rref,w_R,e_is,Ki_s);

== matlab function controlGPI_pos_6dof_conMI/ControladorGPI + NN/Matriz D ==
  data: robot_params input Bus: robot_params_bus; robot_din output Bus: robot_din_bus; q input
function robot_din = fcn(robot_params,q)

robot_din = robot_dinm.din_6dof(robot_params,q,zeros(size(q)));

== matlab function controlGPI_pos_6dof_conMI/Actuadores (Motores de inducción)/MI5 + PBC Torque Controller/Controlador PBC/derivada Corrientes deseadas/derivada Corrientes deseadas ==
  data: MI_motor_params input; d_iSref output size=[2 1]; psi_Rref input size=[2,1]; dpsi_Rref input size=[2,1]; psi_Rmagref input; dpsi_Rmagref input; ddpsi_Rmagref input; tau_Rref input; dtau_Rref input
function d_iSref = fcn(MI_motor_params,psi_Rref,dpsi_Rref,psi_Rmagref,dpsi_Rmagref,ddpsi_Rmagref,tau_Rref,dtau_Rref)

d_iSref = PBC_Torque_Controller.d_iSref(MI_motor_params,psi_Rref,dpsi_Rref,psi_Rmagref,dpsi_Rmagref,ddpsi_Rmagref,tau_Rref,dtau_Rref);

== matlab function controlGPI_pos_6dof_conMI/Actuadores (Motores de inducción)/MI5 + PBC Torque Controller/Modelo MI (Subsistema eléctrico)/Modelo Motor de inducción (Subsistema eléctrico) ==
  data: MI_motor_params input; di_Sab output double size=[2 1]; dpsi_Rab output double size=[2 1]; u_Sab input double size=[2 1]; i_Sab input double size=[2 1]; psi_Rab input double size=[2 1]; w_R input double size=1; tau_R output size=1; tau_L input
function [di_Sab,dpsi_Rab,tau_R] = fcn(MI_motor_params,u_Sab,i_Sab,psi_Rab,w_R,tau_L)

[di_Sab,dpsi_Rab,dw_R,tau_R] = MI_model.MI_space_state(MI_motor_params,u_Sab,i_Sab,psi_Rab,w_R,tau_L);

== matlab function controlGPI_pos_6dof_conMI/Actuadores (Motores de inducción)/MI5 + PBC Torque Controller/Modelo MI (Subsistema eléctrico)/ab//dq ==
  data: psi_ra input; psi_Rmag output; psi_rb input; rho output
function [psi_Rmag,rho] = fcn(psi_ra,psi_rb)

psi_Rmag = sqrt(psi_ra^2+psi_rb^2);
rho = atan2(psi_rb,psi_ra);

== matlab function controlGPI_pos_6dof_conMI/Actuadores (Motores de inducción)/MI6 + PBC Torque Controller/Calculo de Potencia eléctrica/ab0 - ABC ==
  data: BPu input size=[2,1]; u output size=[3,1]
function u = fcn(BPu)

BPu = vertcat(BPu,0);

% Power invariant
BP = transforms.Clarke_transform(1);

u = BP^-1*BPu;

== matlab function controlGPI_pos_6dof_conMI/Actuadores (Motores de inducción)/MI6 + PBC Torque Controller/Calculo de Potencia eléctrica/ab0 - ABC1 ==
  data: BPu input size=[2,1]; u output size=[3,1]
function u = fcn(BPu)

BPu = vertcat(BPu,0);

% Power invariant
BP = transforms.Clarke_transform(1);

u = BP^-1*BPu;

== matlab function controlGPI_pos_6dof_conMI/Actuadores (Motores de inducción)/MI6 + PBC Torque Controller/Controlador PBC/Corrientes y Flujos deseados/Corrientes//Flujos deseados ==
  data: MI_motor_params input; w_R input; i_Sref output size=[2 1]; psi_Rref input size=[2,1]; tau_Rref input; psi_Rmagref input; dpsi_Rmagref input; dpsi_Rref output size=[2,1]
function [i_Sref,dpsi_Rref] = fcn(MI_motor_params,w_R,psi_Rref,tau_Rref,psi_Rmagref,dpsi_Rmagref)

i_Sref = PBC_Torque_Controller.i_Sref(MI_motor_params,psi_Rref,tau_Rref,psi_Rmagref,dpsi_Rmagref);
dpsi_Rref = PBC_Torque_Controller.dpsi_Ref(MI_motor_params,w_R,psi_Rref,tau_Rref,psi_Rmagref,dpsi_Rmagref);

== matlab function controlGPI_pos_6dof_conMI/Actuadores (Motores de inducción)/MI6 + PBC Torque Controller/Controlador PBC/Ley de control/K_iS ==
  data: MI_motor_params input; w_R input; epsilon input; K_iS output
function K_iS = fcn(MI_motor_params,w_R,epsilon)

K_iS = PBC_Torque_Controller.K_iS(MI_motor_params,w_R,epsilon);

== matlab function controlGPI_pos_6dof_conMI/Actuadores (Motores de inducción)/MI6 + PBC Torque Controller/Controlador PBC/Ley de control/Ley de control ==
  data: MI_motor_params input; i_Sref input size=[2,1]; d_iSref input size=[2,1]; u_S output size=[2 1]; psi_Rref input size=[2,1]; w_R input; e_is input; Ki_s input
function u_S = fcn(MI_motor_params,i_Sref,d_iSref,psi_Rref,w_R,e_is,Ki_s)

u_S = PBC_Torque_Controller.ley_control_uS(MI_motor_params,i_Sref,d_iSref,psi_Rref,w_R,e_is,Ki_s);

== matlab function controlGPI_pos_6dof_conMI/Trayectoria de referencia/Inicializar posición de robot manipulador/interp_pol7_q_r ==
  data: t input; q_eq input; interp_qpos output; q_cero input; q_tr_init input; t0 input; t1 input; t_trtr input; tr_muestra input; ndof input
function interp_qpos = fcn(t,q_eq,q_cero,q_tr_init,t0,t1,t_trtr,tr_muestra,ndof)

tcero = t0/2 + t1/2;

if t < tcero
    dist1 = norm(zeros(size(q_eq)) - q_eq);
    
    if dist1 > 0
        qpol1 = pol7(t,0,dist1,t0,tcero);
        dire1 = (zeros(size(q_eq)) - q_eq)/dist1;
        
        interp_qpos = q_eq + dire1*qpol1;
    else
        interp_qpos = q_eq;
    end
elseif t >= tcero && t < t1
    dist2 = norm(q_cero - zeros(size(q_eq)));
    if dist2 > 0
        qpol2 = pol7(t,0,dist2,tcero,t1);
        dire2 = (q_cero - zeros(size(q_eq)))/dist2;
    
        interp_qpos =  zeros(size(q_eq)) + dire2*qpol2;
    else
        interp_qpos = zeros(size(q_eq));
    end
elseif t >= t1 && t < t1 + t_trtr
    if (tr_muestra == 1 || ndof ~= 6) && ndof ~= 2
        dist3 = norm(q_tr_init - q_cero);
        if dist3 > 0
            qpol3 = pol7(t,0,dist3,t1,t1 + t_trtr);
            dire3 = (q_tr_init - q_cero)/dist3;
            
            interp_qpos =  q_cero + dire3*qpol3;
        else
            interp_qpos = q_cero;
        end
    else
        interp_qpos = q_tr_init;
    end
elseif t >= t1 + t_trtr
    interp_qpos = q_tr_init;
else
    interp_qpos = q_eq;
end

== matlab function controlGPI_pos_6dof_conMI/Actuadores (Motores de inducción)/MI6 + PBC Torque Controller/Controlador PBC/derivada Corrientes deseadas/derivada Corrientes deseadas ==
  data: MI_motor_params input; d_iSref output size=[2 1]; psi_Rref input size=[2,1]; dpsi_Rref input size=[2,1]; psi_Rmagref input; dpsi_Rmagref input; ddpsi_Rmagref input; tau_Rref input; dtau_Rref input
function d_iSref = fcn(MI_motor_params,psi_Rref,dpsi_Rref,psi_Rmagref,dpsi_Rmagref,ddpsi_Rmagref,tau_Rref,dtau_Rref)

d_iSref = PBC_Torque_Controller.d_iSref(MI_motor_params,psi_Rref,dpsi_Rref,psi_Rmagref,dpsi_Rmagref,ddpsi_Rmagref,tau_Rref,dtau_Rref);

== matlab function controlGPI_pos_6dof_conMI/Actuadores (Motores de inducción)/MI6 + PBC Torque Controller/Modelo MI (Subsistema eléctrico)/Modelo Motor de inducción (Subsistema eléctrico) ==
  data: MI_motor_params input; di_Sab output double size=[2 1]; dpsi_Rab output double size=[2 1]; u_Sab input double size=[2 1]; i_Sab input double size=[2 1]; psi_Rab input double size=[2 1]; w_R input double size=1; tau_R output size=1; tau_L input
function [di_Sab,dpsi_Rab,tau_R] = fcn(MI_motor_params,u_Sab,i_Sab,psi_Rab,w_R,tau_L)

[di_Sab,dpsi_Rab,dw_R,tau_R] = MI_model.MI_space_state(MI_motor_params,u_Sab,i_Sab,psi_Rab,w_R,tau_L);

== matlab function controlGPI_pos_6dof_conMI/Actuadores (Motores de inducción)/MI6 + PBC Torque Controller/Modelo MI (Subsistema eléctrico)/ab//dq ==
  data: psi_ra input; psi_Rmag output; psi_rb input; rho output
function [psi_Rmag,rho] = fcn(psi_ra,psi_rb)

psi_Rmag = sqrt(psi_ra^2+psi_rb^2);
rho = atan2(psi_rb,psi_ra);

== matlab function controlGPI_pos_6dof_conMI/Actuadores (Motores de inducción)/MI2 + PBC Torque Controller/Controlador PBC/derivada Corrientes deseadas/derivada Corrientes deseadas ==
  data: MI_motor_params input; d_iSref output size=[2 1]; psi_Rref input size=[2,1]; dpsi_Rref input size=[2,1]; psi_Rmagref input; dpsi_Rmagref input; ddpsi_Rmagref input; tau_Rref input; dtau_Rref input
function d_iSref = fcn(MI_motor_params,psi_Rref,dpsi_Rref,psi_Rmagref,dpsi_Rmagref,ddpsi_Rmagref,tau_Rref,dtau_Rref)

d_iSref = PBC_Torque_Controller.d_iSref(MI_motor_params,psi_Rref,dpsi_Rref,psi_Rmagref,dpsi_Rmagref,ddpsi_Rmagref,tau_Rref,dtau_Rref);

== matlab function controlGPI_pos_6dof_conMI/Actuadores (Motores de inducción)/MI2 + PBC Torque Controller/Modelo MI (Subsistema eléctrico)/Modelo Motor de inducción (Subsistema eléctrico) ==
  data: MI_motor_params input; di_Sab output double size=[2 1]; dpsi_Rab output double size=[2 1]; u_Sab input double size=[2 1]; i_Sab input double size=[2 1]; psi_Rab input double size=[2 1]; w_R input double size=1; tau_R output size=1; tau_L input
function [di_Sab,dpsi_Rab,tau_R] = fcn(MI_motor_params,u_Sab,i_Sab,psi_Rab,w_R,tau_L)

[di_Sab,dpsi_Rab,dw_R,tau_R] = MI_model.MI_space_state(MI_motor_params,u_Sab,i_Sab,psi_Rab,w_R,tau_L);

== matlab function controlGPI_pos_6dof_conMI/Actuadores (Motores de inducción)/MI2 + PBC Torque Controller/Modelo MI (Subsistema eléctrico)/ab//dq ==
  data: psi_ra input; psi_Rmag output; psi_rb input; rho output
function [psi_Rmag,rho] = fcn(psi_ra,psi_rb)

psi_Rmag = sqrt(psi_ra^2+psi_rb^2);
rho = atan2(psi_rb,psi_ra);

== matlab function controlGPI_pos_6dof_conMI/Perfil torque de carga tau_L/If Action Subsystem/Senoidal tiempo de inicio ==
  data: t input; tr output; perfil_params input
function tr = fcn(t,perfil_params)

t1 = perfil_params.senoidal.tiempo_inicio;

if t < t1
    tr = 0;
else
    tr = t - t1;
end

== matlab function controlGPI_pos_6dof_conMI/Actuadores (Motores de inducción)/MI3 + PBC Torque Controller/Calculo de Potencia eléctrica/ab0 - ABC ==
  data: BPu input size=[2,1]; u output size=[3,1]
function u = fcn(BPu)

BPu = vertcat(BPu,0);

% Power invariant
BP = transforms.Clarke_transform(1);

u = BP^-1*BPu;

== matlab function controlGPI_pos_6dof_conMI/Norm e_q ==
  data: u input; y output
function y = norm(u)

y = norm(u,2);
